simulink model "node23_case_10kV_withLoad_v2"  (R2022b)
settings: Solver=VariableStepAuto  StartTime=0.0  StopTime=10  FixedStep=1e-6  RelTol=1e-5
InitFcn:
  | sw=5;
  | Lf=1.75e-3+3.5e-3;
  | %Lf=3.5e-3;
  | %Cf=2e-4;
  | f=10;
  | Cf=15e-6;
  | % L=1.75e-3/2;
  | % X=100*pi*L;
  | % R=2*X;
  | R=0.25;X=R/0.66;
  | L=X/100/pi;
  | Z=sqrt(R^2+X^2);
  | f = 30;
  | kp1=10;
  | ki1=100;
  | kp4=20;
  | ki4=100;
  | kp16=20;
  | ki16=100;
  | % 负载参数
  | R1L=0;
  | X1L=0;
  | R2L=652.4467;
  | X2L=276.0351;
  | R3L=804.5741;
  | X3L=256.7790;
  | R4L=760.9867;
  | X4L=234.6376;
  | R5L=818.7384;
  | X5L=266.9799;
  | R6L=671.1329;
  | X6L=170.1801;
  | R7L=883.7621;
  | X7L=178.8663;
  | R8L=388.3725;
  | X8L=158.3040;
  | R9L=817.4819;
  | X9L=268.6933;
  | R10L=849.4733;
  | X10L=254.8420;
  | R11L=407.8415;
  | X11L=165.8504;
  | R12L=NaN;  % Bus 12 无 R、X 数据，用 NaN 标记
  | X12L=NaN;
  | R13L=751.2339;
  | X13L=329.8428;
  | R14L=294.0393;
  | X14L=141.6929;
  | R15L=761.9027;
  | X15L=284.3908;
  | R16L=740.4040;
  | X16L=318.2438;
  | R17L=674.5784;
  | X17L=316.4689;
  | R18L=776.7449;
  | X18L=316.6080;
  | R19L=766.0423;
  | X19L=335.7994;
  | R20L=746.0545;
  | X20L=344.3329;
  | ... (+266 lines)
libraries: spsSeriesRLCBranchLib x210, slpidlib x45, spsControlledVoltageSourceLib x30, spsThreePhaseVIMeasurementLib x24, spsPower3phInstantaneousLib x13, spsAlphaBetaZerotoabcLib x9, spsCurrentMeasurementLib x6, spsGroundLib x2, spspowerguiLib x1
(part 8 of 8)

== matlab function node23_case_10kV_withLoad_v2/IBR-10/IBR1输出电压正负序分离/alphabeta-dq 1 ==
  data: valpha input; vd output; vbeta input; ph input; vq output
function [vd,vq] = fcn(valpha,vbeta,ph)
vd=cos(ph)*valpha+sin(ph)*vbeta;
vq=-sin(ph)*valpha+cos(ph)*vbeta;

== matlab function node23_case_10kV_withLoad_v2/IBR-10/IBR1输出电流正负序分离/abc-alphabeta 1 ==
  data: va input; valpha output; vb input; vc input; vbeta output
function [valpha,vbeta] = fcn(va,vb,vc)
valpha=(2/3)*(1*va-1/2*vb-1/2*vc);
vbeta=(2/3)*(0*va+sqrt(3)/2*vb-sqrt(3)/2*vc);

== matlab function node23_case_10kV_withLoad_v2/IBR-8/MATLAB Function1 ==
  data: u input; y output
function y = fcn(u)
y = rem(u,2*pi);

== matlab function node23_case_10kV_withLoad_v2/IBR-10/IBR1输出电流正负序分离/albe-dq ==
  data: valpha input; vd output; vbeta input; ph input; vq output
function [vd,vq] = fcn(valpha,vbeta,ph)
vd=cos(ph)*valpha+sin(ph)*vbeta;
vq=-sin(ph)*valpha+cos(ph)*vbeta;

== matlab function node23_case_10kV_withLoad_v2/IBR-10/IBR1输出电流正负序分离/alphabeta-dq 1 ==
  data: valpha input; vd output; vbeta input; ph input; vq output
function [vd,vq] = fcn(valpha,vbeta,ph)
vd=cos(ph)*valpha+sin(ph)*vbeta;
vq=-sin(ph)*valpha+cos(ph)*vbeta;

== matlab function node23_case_10kV_withLoad_v2/IBR4/dq轴功率计算 ==
  data: vd_p input; P1 output; vq_p input; vd_n input; vq_n input; id_p input; iq_p input; id_n input; iq_n input; Q1 output; P_p output; P_n output; Q_p output; Q_n output
function [P1, Q1, P_p, P_n, Q_p, Q_n] = fcn(vd_p, vq_p, vd_n, vq_n, id_p, iq_p, id_n, iq_n)
P_p = 1.5*(vd_p*id_p + vq_p*iq_p);
P_n = 1.5*(vd_n*id_n + vq_n*iq_n);
Q_p = 1.5*(vq_p*id_p - vd_p*iq_p);
Q_n = 1.5*(vq_n*id_n - vd_n*iq_n);
P1 = 1.5*(vd_p*id_p + vq_p*iq_p + vd_n*id_n + vq_n*iq_n);
Q1 = 1.5*(vq_p*id_p - vd_p*iq_p + vq_n*id_n - vd_n*iq_n);

%1.5倍

== matlab function node23_case_10kV_withLoad_v2/Grid/negative_sequence_dq>>abc4/MATLAB Function ==
  data: d input; alpha output; q input; theta input; beta output
function [alpha,beta] = fcn(d,q,theta)
%#codegen
A=[cos(theta) sin(theta);
   -sin(theta) cos(theta);];
y = A*[d;q;];
alpha=y(1);
beta=y(2);

== matlab function node23_case_10kV_withLoad_v2/Grid/positive_sequence_dq>>abc1/MATLAB Function ==
  data: d input; alpha output; q input; theta input; beta output
function [alpha,beta] = fcn(d,q,theta)
%#codegen
A=[cos(theta) -sin(theta);
   sin(theta) cos(theta);];
y = A*[d;q;];
alpha=y(1);
beta=y(2);
%alpha轴与A轴重合

== matlab function node23_case_10kV_withLoad_v2/IBR-10/IBR2 ==
  data: vcd_p input; Vc_p output; vcq_p input; vcd_n input; vcq_n input; Vc_n output; VUF output
function [Vc_p, Vc_n, VUF] = fcn(vcd_p, vcq_p, vcd_n, vcq_n)
Vc_p = sqrt(vcd_p^2 + vcq_p^2);
Vc_n = sqrt(vcd_n^2 + vcq_n^2);
VUF = Vc_n/Vc_p;

== matlab function node23_case_10kV_withLoad_v2/T_p1 ==
  data: ud input; Idp output; uq input; ub output; ph input
function [Idp,ub]= fcn(ud,uq,ph)
Idp=ud*cos(ph)+uq*sin(ph);
ub=-ud*sin(ph)+uq*cos(ph);

== matlab function node23_case_10kV_withLoad_v2/IBR-10/MATLAB Function1 ==
  data: u input; y output
function y = fcn(u)
y = rem(u,2*pi);

== matlab function node23_case_10kV_withLoad_v2/IBR-10/MATLAB Function4 ==
  data: ud input; ua output; uq input; ub output; ph input
function [ua,ub]= fcn(ud,uq,ph)
ua=ud*cos(ph)-uq*sin(ph)
ub=ud*sin(ph)+uq*cos(ph)

== matlab function node23_case_10kV_withLoad_v2/IBR-10/MATLAB Function5 ==
  data: ud input; ua output; uq input; ub output; ph input
function [ua,ub]= fcn(ud,uq,ph)
ua=ud*cos(ph)-uq*sin(ph);
ub=ud*sin(ph)+uq*cos(ph);

== matlab function node23_case_10kV_withLoad_v2/IBR-10/abc-alphabeta 10 ==
  data: va input; valpha output; vb input; vc input; vbeta output
function [valpha,vbeta] = fcn(va,vb,vc)
valpha=(2/3)*(1*va-1/2*vb-1/2*vc);
vbeta=(2/3)*(0*va+sqrt(3)/2*vb-sqrt(3)/2*vc);

== matlab function node23_case_10kV_withLoad_v2/IBR-10/albe-dq ==
  data: valpha input; vd output; vbeta input; ph input; vq output
function [vd,vq] = fcn(valpha,vbeta,ph)
vd=cos(ph)*valpha+sin(ph)*vbeta;
vq=-sin(ph)*valpha+cos(ph)*vbeta;

== matlab function node23_case_10kV_withLoad_v2/IBR-10/alphabeta-dq 9 ==
  data: valpha input; vd output; vbeta input; ph input; vq output
function [vd,vq] = fcn(valpha,vbeta,ph)
vd=cos(ph)*valpha+sin(ph)*vbeta;
vq=-sin(ph)*valpha+cos(ph)*vbeta;

== matlab function node23_case_10kV_withLoad_v2/IBR-10/dq轴功率计算 ==
  data: vd_p input; P1 output; vq_p input; vd_n input; vq_n input; id_p input; iq_p input; id_n input; iq_n input; Q1 output; P_p output; P_n output; Q_p output; Q_n output
function [P1, Q1, P_p, P_n, Q_p, Q_n] = fcn(vd_p, vq_p, vd_n, vq_n, id_p, iq_p, id_n, iq_n)
P_p = 1.5*(vd_p*id_p + vq_p*iq_p);
P_n = 1.5*(vd_n*id_n + vq_n*iq_n);
Q_p = 1.5*(vq_p*id_p - vd_p*iq_p);
Q_n = 1.5*(vq_n*id_n - vd_n*iq_n);
P1 = 1.5*(vd_p*id_p + vq_p*iq_p + vd_n*id_n + vq_n*iq_n);
Q1 = 1.5*(vq_p*id_p - vd_p*iq_p + vq_n*id_n - vd_n*iq_n);

%1.5倍

== matlab function node23_case_10kV_withLoad_v2/IBR4/IBR1输出电压正负序分离/abc-alphabeta 1 ==
  data: va input; valpha output; vb input; vc input; vbeta output
function [valpha,vbeta] = fcn(va,vb,vc)
valpha=(2/3)*(1*va-1/2*vb-1/2*vc);
vbeta=(2/3)*(0*va+sqrt(3)/2*vb-sqrt(3)/2*vc);

== matlab function node23_case_10kV_withLoad_v2/IBR4/IBR1输出电压正负序分离/albe-dq ==
  data: valpha input; vd output; vbeta input; ph input; vq output
function [vd,vq] = fcn(valpha,vbeta,ph)
vd=cos(ph)*valpha+sin(ph)*vbeta;
vq=-sin(ph)*valpha+cos(ph)*vbeta;

== matlab function node23_case_10kV_withLoad_v2/IBR-8/abc-alphabeta 10 ==
  data: va input; valpha output; vb input; vc input; vbeta output
function [valpha,vbeta] = fcn(va,vb,vc)
valpha=(2/3)*(1*va-1/2*vb-1/2*vc);
vbeta=(2/3)*(0*va+sqrt(3)/2*vb-sqrt(3)/2*vc);

== matlab function node23_case_10kV_withLoad_v2/IBR4/IBR1输出电压正负序分离/alphabeta-dq 1 ==
  data: valpha input; vd output; vbeta input; ph input; vq output
function [vd,vq] = fcn(valpha,vbeta,ph)
vd=cos(ph)*valpha+sin(ph)*vbeta;
vq=-sin(ph)*valpha+cos(ph)*vbeta;

== matlab function node23_case_10kV_withLoad_v2/IBR4/IBR1输出电流正负序分离/abc-alphabeta 1 ==
  data: va input; valpha output; vb input; vc input; vbeta output
function [valpha,vbeta] = fcn(va,vb,vc)
valpha=(2/3)*(1*va-1/2*vb-1/2*vc);
vbeta=(2/3)*(0*va+sqrt(3)/2*vb-sqrt(3)/2*vc);

== matlab function node23_case_10kV_withLoad_v2/IBR4/IBR1输出电流正负序分离/albe-dq ==
  data: valpha input; vd output; vbeta input; ph input; vq output
function [vd,vq] = fcn(valpha,vbeta,ph)
vd=cos(ph)*valpha+sin(ph)*vbeta;
vq=-sin(ph)*valpha+cos(ph)*vbeta;

== matlab function node23_case_10kV_withLoad_v2/IBR4/IBR1输出电流正负序分离/alphabeta-dq 1 ==
  data: valpha input; vd output; vbeta input; ph input; vq output
function [vd,vq] = fcn(valpha,vbeta,ph)
vd=cos(ph)*valpha+sin(ph)*vbeta;
vq=-sin(ph)*valpha+cos(ph)*vbeta;

== matlab function node23_case_10kV_withLoad_v2/IBR-11/IBR1输出电压正负序分离/abc-alphabeta 1 ==
  data: va input; valpha output; vb input; vc input; vbeta output
function [valpha,vbeta] = fcn(va,vb,vc)
valpha=(2/3)*(1*va-1/2*vb-1/2*vc);
vbeta=(2/3)*(0*va+sqrt(3)/2*vb-sqrt(3)/2*vc);

== matlab function node23_case_10kV_withLoad_v2/IBR-11/IBR1输出电压正负序分离/albe-dq ==
  data: valpha input; vd output; vbeta input; ph input; vq output
function [vd,vq] = fcn(valpha,vbeta,ph)
vd=cos(ph)*valpha+sin(ph)*vbeta;
vq=-sin(ph)*valpha+cos(ph)*vbeta;

== matlab function node23_case_10kV_withLoad_v2/IBR-11/IBR1输出电压正负序分离/alphabeta-dq 1 ==
  data: valpha input; vd output; vbeta input; ph input; vq output
function [vd,vq] = fcn(valpha,vbeta,ph)
vd=cos(ph)*valpha+sin(ph)*vbeta;
vq=-sin(ph)*valpha+cos(ph)*vbeta;

== matlab function node23_case_10kV_withLoad_v2/IBR-11/IBR1输出电流正负序分离/abc-alphabeta 1 ==
  data: va input; valpha output; vb input; vc input; vbeta output
function [valpha,vbeta] = fcn(va,vb,vc)
valpha=(2/3)*(1*va-1/2*vb-1/2*vc);
vbeta=(2/3)*(0*va+sqrt(3)/2*vb-sqrt(3)/2*vc);

== matlab function node23_case_10kV_withLoad_v2/IBR4/MATLAB Function4 ==
  data: ud input; ua output; uq input; ub output; ph input
function [ua,ub]= fcn(ud,uq,ph)
ua=ud*cos(ph)-uq*sin(ph)
ub=ud*sin(ph)+uq*cos(ph)

== matlab function node23_case_10kV_withLoad_v2/IBR4/MATLAB Function5 ==
  data: ud input; ua output; uq input; ub output; ph input
function [ua,ub]= fcn(ud,uq,ph)
ua=ud*cos(ph)-uq*sin(ph);
ub=ud*sin(ph)+uq*cos(ph);

== matlab function node23_case_10kV_withLoad_v2/IBR-8/alphabeta-dq 9 ==
  data: valpha input; vd output; vbeta input; ph input; vq output
function [vd,vq] = fcn(valpha,vbeta,ph)
vd=cos(ph)*valpha+sin(ph)*vbeta;
vq=-sin(ph)*valpha+cos(ph)*vbeta;

== matlab function node23_case_10kV_withLoad_v2/IBR-11/IBR1输出电流正负序分离/albe-dq ==
  data: valpha input; vd output; vbeta input; ph input; vq output
function [vd,vq] = fcn(valpha,vbeta,ph)
vd=cos(ph)*valpha+sin(ph)*vbeta;
vq=-sin(ph)*valpha+cos(ph)*vbeta;

== matlab function node23_case_10kV_withLoad_v2/IBR4/albe-dq ==
  data: valpha input; vd output; vbeta input; ph input; vq output
function [vd,vq] = fcn(valpha,vbeta,ph)
vd=cos(ph)*valpha+sin(ph)*vbeta;
vq=-sin(ph)*valpha+cos(ph)*vbeta;

== matlab function node23_case_10kV_withLoad_v2/IBR-11/IBR1输出电流正负序分离/alphabeta-dq 1 ==
  data: valpha input; vd output; vbeta input; ph input; vq output
function [vd,vq] = fcn(valpha,vbeta,ph)
vd=cos(ph)*valpha+sin(ph)*vbeta;
vq=-sin(ph)*valpha+cos(ph)*vbeta;

== matlab function node23_case_10kV_withLoad_v2/IBR-11/IBR7 ==
  data: vcd_p input; Vc_p output; vcq_p input; vcd_n input; vcq_n input; Vc_n output; VUF output
function [Vc_p, Vc_n, VUF] = fcn(vcd_p, vcq_p, vcd_n, vcq_n)
Vc_p = sqrt(vcd_p^2 + vcq_p^2);
Vc_n = sqrt(vcd_n^2 + vcq_n^2);
VUF = Vc_n/Vc_p;

== matlab function node23_case_10kV_withLoad_v2/IBR-11/MATLAB Function1 ==
  data: u input; y output
function y = fcn(u)
y = rem(u,2*pi);

== matlab function node23_case_10kV_withLoad_v2/IBR-11/MATLAB Function4 ==
  data: ud input; ua output; uq input; ub output; ph input
function [ua,ub]= fcn(ud,uq,ph)
ua=ud*cos(ph)-uq*sin(ph)
ub=ud*sin(ph)+uq*cos(ph)

== matlab function node23_case_10kV_withLoad_v2/IBR-11/MATLAB Function5 ==
  data: ud input; ua output; uq input; ub output; ph input
function [ua,ub]= fcn(ud,uq,ph)
ua=ud*cos(ph)-uq*sin(ph);
ub=ud*sin(ph)+uq*cos(ph);

== matlab function node23_case_10kV_withLoad_v2/IBR-11/abc-alphabeta 10 ==
  data: va input; valpha output; vb input; vc input; vbeta output
function [valpha,vbeta] = fcn(va,vb,vc)
valpha=(2/3)*(1*va-1/2*vb-1/2*vc);
vbeta=(2/3)*(0*va+sqrt(3)/2*vb-sqrt(3)/2*vc);

== matlab function node23_case_10kV_withLoad_v2/IBR-11/albe-dq ==
  data: valpha input; vd output; vbeta input; ph input; vq output
function [vd,vq] = fcn(valpha,vbeta,ph)
vd=cos(ph)*valpha+sin(ph)*vbeta;
vq=-sin(ph)*valpha+cos(ph)*vbeta;

== matlab function node23_case_10kV_withLoad_v2/IBR-11/alphabeta-dq 9 ==
  data: valpha input; vd output; vbeta input; ph input; vq output
function [vd,vq] = fcn(valpha,vbeta,ph)
vd=cos(ph)*valpha+sin(ph)*vbeta;
vq=-sin(ph)*valpha+cos(ph)*vbeta;

== matlab function node23_case_10kV_withLoad_v2/电网电压正负序分离/abc-alphabeta 1 ==
  data: va input; valpha output; vb input; vc input; vbeta output
function [valpha,vbeta] = fcn(va,vb,vc)
valpha=(2/3)*(1*va-1/2*vb-1/2*vc);
vbeta=(2/3)*(0*va+sqrt(3)/2*vb-sqrt(3)/2*vc);

== matlab function node23_case_10kV_withLoad_v2/IBR-11/dq轴功率计算 ==
  data: vd_p input; P1 output; vq_p input; vd_n input; vq_n input; id_p input; iq_p input; id_n input; iq_n input; Q1 output; P_p output; P_n output; Q_p output; Q_n output
function [P1, Q1, P_p, P_n, Q_p, Q_n] = fcn(vd_p, vq_p, vd_n, vq_n, id_p, iq_p, id_n, iq_n)
P_p = 1.5*(vd_p*id_p + vq_p*iq_p);
P_n = 1.5*(vd_n*id_n + vq_n*iq_n);
Q_p = 1.5*(vq_p*id_p - vd_p*iq_p);
Q_n = 1.5*(vq_n*id_n - vd_n*iq_n);
P1 = 1.5*(vd_p*id_p + vq_p*iq_p + vd_n*id_n + vq_n*iq_n);
Q1 = 1.5*(vq_p*id_p - vd_p*iq_p + vq_n*id_n - vd_n*iq_n);

%1.5倍

== matlab function node23_case_10kV_withLoad_v2/IBR-12/IBR1输出电压正负序分离/abc-alphabeta 1 ==
  data: va input; valpha output; vb input; vc input; vbeta output
function [valpha,vbeta] = fcn(va,vb,vc)
valpha=(2/3)*(1*va-1/2*vb-1/2*vc);
vbeta=(2/3)*(0*va+sqrt(3)/2*vb-sqrt(3)/2*vc);

== matlab function node23_case_10kV_withLoad_v2/IBR-12/IBR1输出电压正负序分离/albe-dq ==
  data: valpha input; vd output; vbeta input; ph input; vq output
function [vd,vq] = fcn(valpha,vbeta,ph)
vd=cos(ph)*valpha+sin(ph)*vbeta;
vq=-sin(ph)*valpha+cos(ph)*vbeta;

== matlab function node23_case_10kV_withLoad_v2/IBR-8/IBR1输出电压正负序分离/abc-alphabeta 1 ==
  data: va input; valpha output; vb input; vc input; vbeta output
function [valpha,vbeta] = fcn(va,vb,vc)
valpha=(2/3)*(1*va-1/2*vb-1/2*vc);
vbeta=(2/3)*(0*va+sqrt(3)/2*vb-sqrt(3)/2*vc);

== matlab function node23_case_10kV_withLoad_v2/IBR-8/IBR1输出电压正负序分离/albe-dq ==
  data: valpha input; vd output; vbeta input; ph input; vq output
function [vd,vq] = fcn(valpha,vbeta,ph)
vd=cos(ph)*valpha+sin(ph)*vbeta;
vq=-sin(ph)*valpha+cos(ph)*vbeta;

== matlab function node23_case_10kV_withLoad_v2/IBR-8/IBR1输出电压正负序分离/alphabeta-dq 1 ==
  data: valpha input; vd output; vbeta input; ph input; vq output
function [vd,vq] = fcn(valpha,vbeta,ph)
vd=cos(ph)*valpha+sin(ph)*vbeta;
vq=-sin(ph)*valpha+cos(ph)*vbeta;

== matlab function node23_case_10kV_withLoad_v2/IBR-8/IBR1输出电流正负序分离/abc-alphabeta 1 ==
  data: va input; valpha output; vb input; vc input; vbeta output
function [valpha,vbeta] = fcn(va,vb,vc)
valpha=(2/3)*(1*va-1/2*vb-1/2*vc);
vbeta=(2/3)*(0*va+sqrt(3)/2*vb-sqrt(3)/2*vc);

== matlab function node23_case_10kV_withLoad_v2/IBR-8/IBR1输出电流正负序分离/albe-dq ==
  data: valpha input; vd output; vbeta input; ph input; vq output
function [vd,vq] = fcn(valpha,vbeta,ph)
vd=cos(ph)*valpha+sin(ph)*vbeta;
vq=-sin(ph)*valpha+cos(ph)*vbeta;

== matlab function node23_case_10kV_withLoad_v2/IBR-8/IBR1输出电流正负序分离/alphabeta-dq 1 ==
  data: valpha input; vd output; vbeta input; ph input; vq output
function [vd,vq] = fcn(valpha,vbeta,ph)
vd=cos(ph)*valpha+sin(ph)*vbeta;
vq=-sin(ph)*valpha+cos(ph)*vbeta;

== matlab function node23_case_10kV_withLoad_v2/电网电压正负序分离/albe-dq ==
  data: valpha input; vd output; vbeta input; ph input; vq output
function [vd,vq] = fcn(valpha,vbeta,ph)
vd=cos(ph)*valpha+sin(ph)*vbeta;
vq=-sin(ph)*valpha+cos(ph)*vbeta;

== matlab function node23_case_10kV_withLoad_v2/IBR-8/IBR7 ==
  data: vcd_p input; Vc_p output; vcq_p input; vcd_n input; vcq_n input; Vc_n output; VUF output
function [Vc_p, Vc_n, VUF] = fcn(vcd_p, vcq_p, vcd_n, vcq_n)
Vc_p = sqrt(vcd_p^2 + vcq_p^2);
Vc_n = sqrt(vcd_n^2 + vcq_n^2);
VUF = Vc_n/Vc_p;

== matlab function node23_case_10kV_withLoad_v2/IBR-8/MATLAB Function4 ==
  data: ud input; ua output; uq input; ub output; ph input
function [ua,ub]= fcn(ud,uq,ph)
ua=ud*cos(ph)-uq*sin(ph)
ub=ud*sin(ph)+uq*cos(ph)

== matlab function node23_case_10kV_withLoad_v2/IBR-8/MATLAB Function5 ==
  data: ud input; ua output; uq input; ub output; ph input
function [ua,ub]= fcn(ud,uq,ph)
ua=ud*cos(ph)-uq*sin(ph);
ub=ud*sin(ph)+uq*cos(ph);

== matlab function node23_case_10kV_withLoad_v2/IBR-12/IBR1输出电压正负序分离/alphabeta-dq 1 ==
  data: valpha input; vd output; vbeta input; ph input; vq output
function [vd,vq] = fcn(valpha,vbeta,ph)
vd=cos(ph)*valpha+sin(ph)*vbeta;
vq=-sin(ph)*valpha+cos(ph)*vbeta;

== matlab function node23_case_10kV_withLoad_v2/IBR-8/albe-dq ==
  data: valpha input; vd output; vbeta input; ph input; vq output
function [vd,vq] = fcn(valpha,vbeta,ph)
vd=cos(ph)*valpha+sin(ph)*vbeta;
vq=-sin(ph)*valpha+cos(ph)*vbeta;

== matlab function node23_case_10kV_withLoad_v2/IBR-8/dq轴功率计算 ==
  data: vd_p input; P1 output; vq_p input; vd_n input; vq_n input; id_p input; iq_p input; id_n input; iq_n input; Q1 output; P_p output; P_n output; Q_p output; Q_n output
function [P1, Q1, P_p, P_n, Q_p, Q_n] = fcn(vd_p, vq_p, vd_n, vq_n, id_p, iq_p, id_n, iq_n)
P_p = 1.5*(vd_p*id_p + vq_p*iq_p);
P_n = 1.5*(vd_n*id_n + vq_n*iq_n);
Q_p = 1.5*(vq_p*id_p - vd_p*iq_p);
Q_n = 1.5*(vq_n*id_n - vd_n*iq_n);
P1 = 1.5*(vd_p*id_p + vq_p*iq_p + vd_n*id_n + vq_n*iq_n);
Q1 = 1.5*(vq_p*id_p - vd_p*iq_p + vq_n*id_n - vd_n*iq_n);

%1.5倍

== matlab function node23_case_10kV_withLoad_v2/IBR-12/IBR1输出电流正负序分离/abc-alphabeta 1 ==
  data: va input; valpha output; vb input; vc input; vbeta output
function [valpha,vbeta] = fcn(va,vb,vc)
valpha=(2/3)*(1*va-1/2*vb-1/2*vc);
vbeta=(2/3)*(0*va+sqrt(3)/2*vb-sqrt(3)/2*vc);

== matlab function node23_case_10kV_withLoad_v2/IBR-12/IBR1输出电流正负序分离/albe-dq ==
  data: valpha input; vd output; vbeta input; ph input; vq output
function [vd,vq] = fcn(valpha,vbeta,ph)
vd=cos(ph)*valpha+sin(ph)*vbeta;
vq=-sin(ph)*valpha+cos(ph)*vbeta;

== matlab function node23_case_10kV_withLoad_v2/IBR-12/IBR1输出电流正负序分离/alphabeta-dq 1 ==
  data: valpha input; vd output; vbeta input; ph input; vq output
function [vd,vq] = fcn(valpha,vbeta,ph)
vd=cos(ph)*valpha+sin(ph)*vbeta;
vq=-sin(ph)*valpha+cos(ph)*vbeta;

== matlab function node23_case_10kV_withLoad_v2/IBR4/IBR2 ==
  data: vcd_p input; Vc_p output; vcq_p input; vcd_n input; vcq_n input; Vc_n output; VUF output
function [Vc_p, Vc_n, VUF] = fcn(vcd_p, vcq_p, vcd_n, vcq_n)
Vc_p = sqrt(vcd_p^2 + vcq_p^2);
Vc_n = sqrt(vcd_n^2 + vcq_n^2);
VUF = Vc_n/Vc_p;

== matlab function node23_case_10kV_withLoad_v2/IBR-12/IBR7 ==
  data: vcd_p input; Vc_p output; vcq_p input; vcd_n input; vcq_n input; Vc_n output; VUF output
function [Vc_p, Vc_n, VUF] = fcn(vcd_p, vcq_p, vcd_n, vcq_n)
Vc_p = sqrt(vcd_p^2 + vcq_p^2);
Vc_n = sqrt(vcd_n^2 + vcq_n^2);
VUF = Vc_n/Vc_p;

== matlab function node23_case_10kV_withLoad_v2/IBR-12/MATLAB Function1 ==
  data: u input; y output
function y = fcn(u)
y = rem(u,2*pi);

== matlab function node23_case_10kV_withLoad_v2/IBR-12/MATLAB Function4 ==
  data: ud input; ua output; uq input; ub output; ph input
function [ua,ub]= fcn(ud,uq,ph)
ua=ud*cos(ph)-uq*sin(ph)
ub=ud*sin(ph)+uq*cos(ph)

== matlab function node23_case_10kV_withLoad_v2/IBR-12/MATLAB Function5 ==
  data: ud input; ua output; uq input; ub output; ph input
function [ua,ub]= fcn(ud,uq,ph)
ua=ud*cos(ph)-uq*sin(ph);
ub=ud*sin(ph)+uq*cos(ph);

== matlab function node23_case_10kV_withLoad_v2/IBR-12/abc-alphabeta 10 ==
  data: va input; valpha output; vb input; vc input; vbeta output
function [valpha,vbeta] = fcn(va,vb,vc)
valpha=(2/3)*(1*va-1/2*vb-1/2*vc);
vbeta=(2/3)*(0*va+sqrt(3)/2*vb-sqrt(3)/2*vc);

== matlab function node23_case_10kV_withLoad_v2/IBR-12/albe-dq ==
  data: valpha input; vd output; vbeta input; ph input; vq output
function [vd,vq] = fcn(valpha,vbeta,ph)
vd=cos(ph)*valpha+sin(ph)*vbeta;
vq=-sin(ph)*valpha+cos(ph)*vbeta;

== matlab function node23_case_10kV_withLoad_v2/IBR-12/alphabeta-dq 9 ==
  data: valpha input; vd output; data output; vbeta input; ph input; vq output
function [vd,data, vq] = fcn(valpha,vbeta,ph)
vd=cos(ph)*valpha+sin(ph)*vbeta;
vq=-sin(ph)*valpha+cos(ph)*vbeta;

== matlab function node23_case_10kV_withLoad_v2/IBR-12/dq轴功率计算 ==
  data: vd_p input; P1 output; vq_p input; vd_n input; vq_n input; id_p input; iq_p input; id_n input; iq_n input; Q1 output; P_p output; P_n output; Q_p output; Q_n output
function [P1, Q1, P_p, P_n, Q_p, Q_n] = fcn(vd_p, vq_p, vd_n, vq_n, id_p, iq_p, id_n, iq_n)
P_p = 1.5*(vd_p*id_p + vq_p*iq_p);
P_n = 1.5*(vd_n*id_n + vq_n*iq_n);
Q_p = 1.5*(vq_p*id_p - vd_p*iq_p);
Q_n = 1.5*(vq_n*id_n - vd_n*iq_n);
P1 = 1.5*(vd_p*id_p + vq_p*iq_p + vd_n*id_n + vq_n*iq_n);
Q1 = 1.5*(vq_p*id_p - vd_p*iq_p + vq_n*id_n - vd_n*iq_n);

%1.5倍

== matlab function node23_case_10kV_withLoad_v2/IBR-16/IBR1输出电压正负序分离/abc-alphabeta 1 ==
  data: va input; valpha output; vb input; vc input; vbeta output
function [valpha,vbeta] = fcn(va,vb,vc)
valpha=(2/3)*(1*va-1/2*vb-1/2*vc);
vbeta=(2/3)*(0*va+sqrt(3)/2*vb-sqrt(3)/2*vc);

== matlab function node23_case_10kV_withLoad_v2/IBR-16/IBR1输出电压正负序分离/albe-dq ==
  data: valpha input; vd output; vbeta input; ph input; vq output
function [vd,vq] = fcn(valpha,vbeta,ph)
vd=cos(ph)*valpha+sin(ph)*vbeta;
vq=-sin(ph)*valpha+cos(ph)*vbeta;

== matlab function node23_case_10kV_withLoad_v2/IBR-16/IBR1输出电压正负序分离/alphabeta-dq 1 ==
  data: valpha input; vd output; vbeta input; ph input; vq output
function [vd,vq] = fcn(valpha,vbeta,ph)
vd=cos(ph)*valpha+sin(ph)*vbeta;
vq=-sin(ph)*valpha+cos(ph)*vbeta;

== matlab function node23_case_10kV_withLoad_v2/电网电压正负序分离/alphabeta-dq 1 ==
  data: valpha input; vd output; vbeta input; ph input; vq output
function [vd,vq] = fcn(valpha,vbeta,ph)
vd=cos(ph)*valpha+sin(ph)*vbeta;
vq=-sin(ph)*valpha+cos(ph)*vbeta;

== matlab function node23_case_10kV_withLoad_v2/IBR-16/IBR1输出电流正负序分离/abc-alphabeta 1 ==
  data: va input; valpha output; vb input; vc input; vbeta output
function [valpha,vbeta] = fcn(va,vb,vc)
valpha=(2/3)*(1*va-1/2*vb-1/2*vc);
vbeta=(2/3)*(0*va+sqrt(3)/2*vb-sqrt(3)/2*vc);

== matlab function node23_case_10kV_withLoad_v2/IBR-16/IBR1输出电流正负序分离/albe-dq ==
  data: valpha input; vd output; vbeta input; ph input; vq output
function [vd,vq] = fcn(valpha,vbeta,ph)
vd=cos(ph)*valpha+sin(ph)*vbeta;
vq=-sin(ph)*valpha+cos(ph)*vbeta;

== matlab function node23_case_10kV_withLoad_v2/IBR-16/IBR1输出电流正负序分离/alphabeta-dq 1 ==
  data: valpha input; vd output; vbeta input; ph input; vq output
function [vd,vq] = fcn(valpha,vbeta,ph)
vd=cos(ph)*valpha+sin(ph)*vbeta;
vq=-sin(ph)*valpha+cos(ph)*vbeta;

== matlab function node23_case_10kV_withLoad_v2/IBR-16/IBR7 ==
  data: vcd_p input; Vc_p output; vcq_p input; vcd_n input; vcq_n input; Vc_n output; VUF output
function [Vc_p, Vc_n, VUF] = fcn(vcd_p, vcq_p, vcd_n, vcq_n)
Vc_p = sqrt(vcd_p^2 + vcq_p^2);
Vc_n = sqrt(vcd_n^2 + vcq_n^2);
VUF = Vc_n/Vc_p;

== matlab function node23_case_10kV_withLoad_v2/IBR-16/MATLAB Function1 ==
  data: u input; y output
function y = fcn(u)
y = rem(u,2*pi);

== matlab function node23_case_10kV_withLoad_v2/IBR-16/MATLAB Function4 ==
  data: ud input; ua output; uq input; ub output; ph input
function [ua,ub]= fcn(ud,uq,ph)
ua=ud*cos(ph)-uq*sin(ph)
ub=ud*sin(ph)+uq*cos(ph)

== matlab function node23_case_10kV_withLoad_v2/IBR-16/MATLAB Function5 ==
  data: ud input; ua output; uq input; ub output; ph input
function [ua,ub]= fcn(ud,uq,ph)
ua=ud*cos(ph)-uq*sin(ph);
ub=ud*sin(ph)+uq*cos(ph);

== matlab function node23_case_10kV_withLoad_v2/IBR-16/abc-alphabeta 10 ==
  data: va input; valpha output; vb input; vc input; vbeta output
function [valpha,vbeta] = fcn(va,vb,vc)
valpha=(2/3)*(1*va-1/2*vb-1/2*vc);
vbeta=(2/3)*(0*va+sqrt(3)/2*vb-sqrt(3)/2*vc);

== matlab function node23_case_10kV_withLoad_v2/IBR-16/albe-dq ==
  data: valpha input; vd output; vbeta input; ph input; vq output
function [vd,vq] = fcn(valpha,vbeta,ph)
vd=cos(ph)*valpha+sin(ph)*vbeta;
vq=-sin(ph)*valpha+cos(ph)*vbeta;

== matlab function node23_case_10kV_withLoad_v2/IBR-16/alphabeta-dq 9 ==
  data: valpha input; vd output; vbeta input; ph input; vq output
function [vd,vq] = fcn(valpha,vbeta,ph)
vd=cos(ph)*valpha+sin(ph)*vbeta;
vq=-sin(ph)*valpha+cos(ph)*vbeta;

== matlab function node23_case_10kV_withLoad_v2/IBR-16/dq轴功率计算 ==
  data: vd_p input; P1 output; vq_p input; vd_n input; vq_n input; id_p input; iq_p input; id_n input; iq_n input; Q1 output; P_p output; P_n output; Q_p output; Q_n output
function [P1, Q1, P_p, P_n, Q_p, Q_n] = fcn(vd_p, vq_p, vd_n, vq_n, id_p, iq_p, id_n, iq_n)
P_p = 1.5*(vd_p*id_p + vq_p*iq_p);
P_n = 1.5*(vd_n*id_n + vq_n*iq_n);
Q_p = 1.5*(vq_p*id_p - vd_p*iq_p);
Q_n = 1.5*(vq_n*id_n - vd_n*iq_n);
P1 = 1.5*(vd_p*id_p + vq_p*iq_p + vd_n*id_n + vq_n*iq_n);
Q1 = 1.5*(vq_p*id_p - vd_p*iq_p + vq_n*id_n - vd_n*iq_n);

%1.5倍

== matlab function node23_case_10kV_withLoad_v2/T_p7 ==
  data: ud input; Idp output; uq input; ub output; ph input
function [Idp,ub]= fcn(ud,uq,ph)
Idp=ud*cos(ph)+uq*sin(ph);
ub=-ud*sin(ph)+uq*cos(ph);

== matlab function node23_case_10kV_withLoad_v2/IBR-21/IBR1输出电压正负序分离/abc-alphabeta 1 ==
  data: va input; valpha output; vb input; vc input; vbeta output
function [valpha,vbeta] = fcn(va,vb,vc)
valpha=(2/3)*(1*va-1/2*vb-1/2*vc);
vbeta=(2/3)*(0*va+sqrt(3)/2*vb-sqrt(3)/2*vc);
